simulink model "akz_ab2"  (Simulink 4.00)
settings: Solver=ode23  SolverMode=SingleTasking  StartTime=0.0  StopTime=80  RelTol=1e-4  AbsTol=1e-8
libraries: simulink3 x1
CloseFcn:
  | ;slview('closediagram',bdroot);
settings Model: LimitDataPoints=off  BlockReductionOpt=off

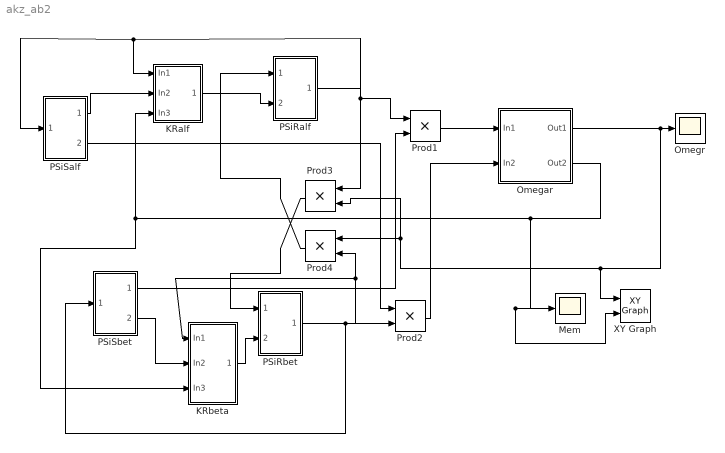
== system akz_ab2 ==
  "  Prod1" : Product  Inputs=2  Multiplication=Element-wise(.*)  SaturateOnIntegerOverflow=on
  KRalf : Subsystem
      settings: RTWFcnNameOpts=Auto  RTWFileNameOpts=Auto
  KRbeta : Subsystem
      settings: RTWFcnNameOpts=Auto  RTWFileNameOpts=Auto
  Mem : Scope
      settings: TickLabels=on  TimeRange=80  YMin=-1  YMax=2  SaveToWorkspace=off  SaveName=ScopeData  DataFormat=Array  MaxDataPoints=5000
  Omegar : Subsystem
      settings: RTWFcnNameOpts=Auto  RTWFileNameOpts=Auto
  Omegr : Scope
      settings: TickLabels=on  TimeRange=80  YMin=0  YMax=1.4  SaveToWorkspace=off  DataFormat=Array  MaxDataPoints=5000
  PSiRalf : Subsystem
      settings: RTWFcnNameOpts=Auto  RTWFileNameOpts=Auto
  PSiRbet : Subsystem
      settings: RTWFcnNameOpts=Auto  RTWFileNameOpts=Auto
  PSiSalf : Subsystem
      settings: RTWFcnNameOpts=Auto  RTWFileNameOpts=Auto
  PSiSbet : Subsystem
      settings: RTWFcnNameOpts=Auto  RTWFileNameOpts=Auto
  Prod2 : Product  Inputs=2  Multiplication=Element-wise(.*)  SaturateOnIntegerOverflow=on
  Prod3 : Product  Orientation=left  Inputs=2  Multiplication=Element-wise(.*)  SaturateOnIntegerOverflow=on
  Prod4 : Product  Orientation=left  Inputs=2  Multiplication=Element-wise(.*)  SaturateOnIntegerOverflow=on
  XY Graph : simulink3/Sinks/XY Graph  xmin=-0.1  xmax=1.2  ymin=-0.1  ymax=1.8  st=-1
  wires:
  Prod2/1 -> Omegar/2(In2)
  "  Prod1"/1 -> Omegar/1(In1)
  Prod4/1 -> PSiRalf/1(In1)
  Prod3/1 -> PSiRbet/1(In1)
  Omegar/1(Out1) -> Omegr/1, Prod4/1, Prod3/2, XY Graph/1
  PSiSalf/2(Out2) -> Prod2/1
  PSiSbet/1(Out1) -> "  Prod1"/2
  Omegar/2(Out2) -> Mem/1, XY Graph/2, KRalf/3(In3), KRbeta/3(In3)
  PSiRbet/1(Out1) -> Prod2/2, PSiSbet/1(In1), Prod4/2, KRbeta/1(In1)
  PSiRalf/1(Out1) -> Prod3/1, "  Prod1"/1, PSiSalf/1(In1), KRalf/1(In1)
  PSiSalf/1(Out1) -> KRalf/2(In2)
  KRbeta/1(Out1) -> PSiRbet/2(In2)
  PSiSbet/2(Out2) -> KRbeta/2(In2)
  KRalf/1(Out1) -> PSiRalf/2(In2)

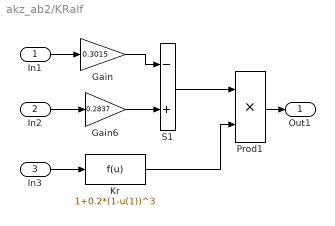
== system akz_ab2/KRalf ==
  In1 : Inport  Port=1
  In2 : Inport  Port=2
  In3 : Inport  Port=3
  "  Prod1" : Product  Inputs=2  Multiplication=Element-wise(.*)  SaturateOnIntegerOverflow=on
  Gain : Gain  Gain=0.3015  Multiplication=Element-wise(K.*u)  SaturateOnIntegerOverflow=on
  Gain6 : Gain  Gain=0.2837  Multiplication=Element-wise(K.*u)  SaturateOnIntegerOverflow=on
  Kr : Fcn  Expr=1+0.2*(1-u(1))^3
  S1 : Sum  Inputs=-+  SaturateOnIntegerOverflow=on
  Out1 : Outport  Port=1
  wires:
  Gain/1 -> S1/1
  Gain6/1 -> S1/2
  In1/1 -> Gain/1
  In2/1 -> Gain6/1
  Kr/1 -> "  Prod1"/2
  S1/1 -> "  Prod1"/1
  "  Prod1"/1 -> Out1/1
  In3/1 -> Kr/1

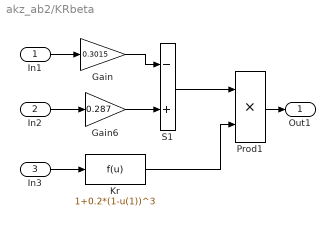
== system akz_ab2/KRbeta ==
  In1 : Inport  Port=1
  In2 : Inport  Port=2
  In3 : Inport  Port=3
  "  Prod1" : Product  Inputs=2  Multiplication=Element-wise(.*)  SaturateOnIntegerOverflow=on
  Gain : Gain  Gain=0.3015  Multiplication=Element-wise(K.*u)  SaturateOnIntegerOverflow=on
  Gain6 : Gain  Gain=0.287  Multiplication=Element-wise(K.*u)  SaturateOnIntegerOverflow=on
  Kr : Fcn  Expr=1+0.2*(1-u(1))^3
  S1 : Sum  Inputs=-+  SaturateOnIntegerOverflow=on
  Out1 : Outport  Port=1
  wires:
  Gain/1 -> S1/1
  Gain6/1 -> S1/2
  In1/1 -> Gain/1
  In2/1 -> Gain6/1
  Kr/1 -> "  Prod1"/2
  S1/1 -> "  Prod1"/1
  "  Prod1"/1 -> Out1/1
  In3/1 -> Kr/1

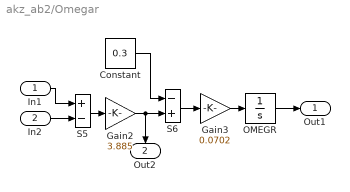
== system akz_ab2/Omegar ==
  In1 : Inport  Port=1
  In2 : Inport  Port=2
  Constant : Constant  Value=0.3
  Gain2 : Gain  Gain=3.885  Multiplication=Element-wise(K.*u)  SaturateOnIntegerOverflow=on
  Gain3 : Gain  Gain=0.0702  Multiplication=Element-wise(K.*u)  SaturateOnIntegerOverflow=on
  OMEGR : Integrator  ExternalReset=none  InitialConditionSource=internal  InitialCondition=0  LimitOutput=off  UpperSaturationLimit=inf  LowerSaturationLimit=-inf  ShowSaturationPort=off  ShowStatePort=off  AbsoluteTolerance=auto
  S5 : Sum  Inputs=+-  SaturateOnIntegerOverflow=on
  S6 : Sum  Inputs=-+  SaturateOnIntegerOverflow=on
  Out1 : Outport  Port=1
  Out2 : Outport  Orientation=down  Port=2
  wires:
  S6/1 -> Gain3/1
  Gain3/1 -> OMEGR/1
  Constant/1 -> S6/1
  S5/1 -> Gain2/1
  Gain2/1 -> S6/2, Out2/1
  In1/1 -> S5/1
  OMEGR/1 -> Out1/1
  In2/1 -> S5/2

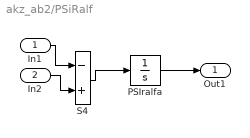
== system akz_ab2/PSiRalf ==
  In1 : Inport  Port=1
  In2 : Inport  Port=2
  PSIralfa : Integrator  ExternalReset=none  InitialConditionSource=internal  InitialCondition=0  LimitOutput=off  UpperSaturationLimit=inf  LowerSaturationLimit=-inf  ShowSaturationPort=off  ShowStatePort=off  AbsoluteTolerance=auto
  S4 : Sum  Inputs=-+  SaturateOnIntegerOverflow=on
  Out1 : Outport  Port=1
  wires:
  In2/1 -> S4/2
  In1/1 -> S4/1
  S4/1 -> PSIralfa/1
  PSIralfa/1 -> Out1/1

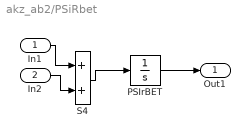
== system akz_ab2/PSiRbet ==
  In1 : Inport  Port=1
  In2 : Inport  Port=2
  PSIrBET : Integrator  ExternalReset=none  InitialConditionSource=internal  InitialCondition=0  LimitOutput=off  UpperSaturationLimit=inf  LowerSaturationLimit=-inf  ShowSaturationPort=off  ShowStatePort=off  AbsoluteTolerance=auto
  S4 : Sum  Inputs=++  SaturateOnIntegerOverflow=on
  Out1 : Outport  Port=1
  wires:
  PSIrBET/1 -> Out1/1
  S4/1 -> PSIrBET/1
  In1/1 -> S4/1
  In2/1 -> S4/2

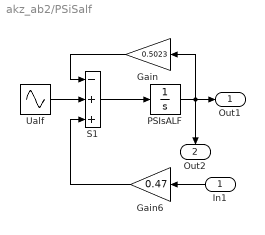
== system akz_ab2/PSiSalf ==
  In1 : Inport  Orientation=left  Port=1
  Gain : Gain  Orientation=left  Gain=0.5023  Multiplication=Element-wise(K.*u)  SaturateOnIntegerOverflow=on
  Gain6 : Gain  Orientation=left  Gain=0.47  Multiplication=Element-wise(K.*u)  SaturateOnIntegerOverflow=on
  PSIsALF : Integrator  ExternalReset=none  InitialConditionSource=internal  InitialCondition=0  LimitOutput=off  UpperSaturationLimit=inf  LowerSaturationLimit=-inf  ShowSaturationPort=off  ShowStatePort=off  AbsoluteTolerance=auto
  S1 : Sum  Inputs=-++  SaturateOnIntegerOverflow=on
  Ualf : Sin  Amplitude=1  Frequency=1  Phase=pi/2  SampleTime=0
  Out1 : Outport  Port=1
  Out2 : Outport  Orientation=down  Port=2
  wires:
  Gain/1 -> S1/1
  S1/1 -> PSIsALF/1
  PSIsALF/1 -> Gain/1, Out1/1, Out2/1
  Ualf/1 -> S1/2
  Gain6/1 -> S1/3
  In1/1 -> Gain6/1

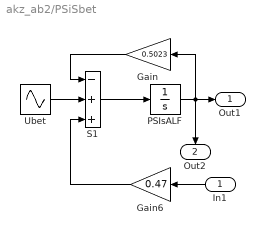
== system akz_ab2/PSiSbet ==
  In1 : Inport  Orientation=left  Port=1
  Gain : Gain  Orientation=left  Gain=0.5023  Multiplication=Element-wise(K.*u)  SaturateOnIntegerOverflow=on
  Gain6 : Gain  Orientation=left  Gain=0.47  Multiplication=Element-wise(K.*u)  SaturateOnIntegerOverflow=on
  PSIsALF : Integrator  ExternalReset=none  InitialConditionSource=internal  InitialCondition=0  LimitOutput=off  UpperSaturationLimit=inf  LowerSaturationLimit=-inf  ShowSaturationPort=off  ShowStatePort=off  AbsoluteTolerance=auto
  S1 : Sum  Inputs=-++  SaturateOnIntegerOverflow=on
  Ubet : Sin  Amplitude=1  Frequency=1  Phase=0  SampleTime=0
  Out1 : Outport  Port=1
  Out2 : Outport  Orientation=down  Port=2
  wires:
  In1/1 -> Gain6/1
  Gain6/1 -> S1/3
  Ubet/1 -> S1/2
  PSIsALF/1 -> Out2/1, Out1/1, Gain/1
  S1/1 -> PSIsALF/1
  Gain/1 -> S1/1
